simulink model "simulink"  (R2022b)
settings: Solver=VariableStepAuto  StartTime=0.0  StopTime=20.0  RelTol=1e-3
values from neighbouring files (symbols this model uses):
  Kp = 10.8    [simulink_data.m]
  Td = 0.27625    [simulink_data.m]
  Ti = 1.105    [simulink_data.m]
settings Model: Creator=parince  LastModifiedBy=parince

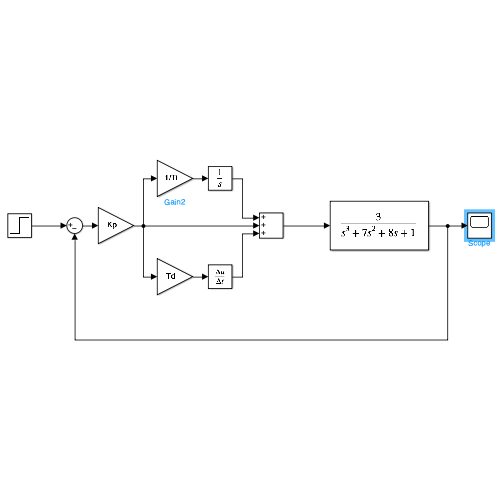
[thumbnail: Simulink's stored preview of the top-level diagram]
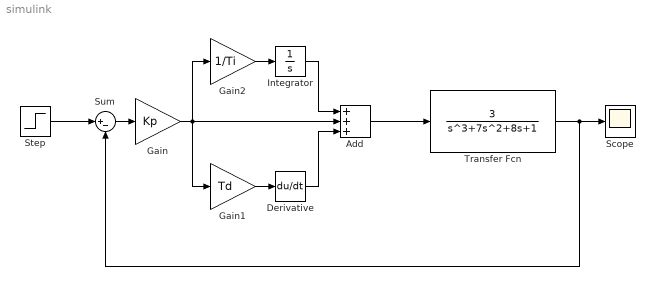
== system simulink ==
  Add : Sum  Inputs=+++
  Derivative : Derivative
  Gain : Gain  Gain=Kp
  Gain1 : Gain  Gain=Td
  Gain2 : Gain  Gain=1/Ti
  Integrator : Integrator
  Scope : Scope
  Step : Step  SampleTime=0
  Sum : Sum  Inputs=|+-
  Transfer Fcn : TransferFcn  Numerator=[3]  Denominator=[1 7 8 1]
  wires:
  Step/1 -> Sum/1
  Sum/1 -> Gain/1
  Gain/1 -> Gain2/1, Gain1/1, Add/2
  Gain2/1 -> Integrator/1
  Gain1/1 -> Derivative/1
  Integrator/1 -> Add/1
  Derivative/1 -> Add/3
  Add/1 -> Transfer Fcn/1
  Transfer Fcn/1 -> Sum/2, Scope/1
